simulink library "Source_Lib"  (R2021a)
settings: Solver=VariableStepAuto  StartTime=0.0  StopTime=10.0  RelTol=1e-3
undefined symbols (not defined in the file or in its folder): Cmu0, delta0, fb, GOV1_K2, ia0, ib0, ic0, pha0, phb0, phc0, Theta0_deg, Time_Step, V0_pu, Vfu0
libraries: spsBreakerLib x12, spsControlledVoltageSourceLib x6, spsThreePhaseSourceLib x5, Control_Lib x4, spsThreePhaseVIMeasurementLib x3, spsSeriesRLCBranchLib x2, spsDCVoltageSourceLib x2, spsGroundLib x2, spsLoadFlowBusLib x2, spsThreePhaseParallelRLCLoadLib x1, spsThreePhaseTransformerTwoWindingsLib x1, spsPower3phInstantaneousLib x1
(part 2 of 2)

== system Source_Lib/Generic Voltage Source old/Source_For_OP ==
  v_abc_ref : Inport
  Controlled Voltage Source1 : spsControlledVoltageSourceLib/Controlled Voltage Source  Initialize=off  Source_Type=AC  Amplitude=V0*Ub*sqrt(2/3)*sin(Theta0)  Phase=(Theta0*180/pi)  Frequency=fb  Measurements=None
  Controlled Voltage Source2 : spsControlledVoltageSourceLib/Controlled Voltage Source  Initialize=off  Source_Type=AC  Amplitude=V0*Ub*sqrt(2/3)*sin(Theta0-2*pi/3)  Phase=(Theta0*180/pi)-120  Frequency=fb  Measurements=None
  Controlled Voltage Source3 : spsControlledVoltageSourceLib/Controlled Voltage Source  Initialize=off  Source_Type=AC  Amplitude=V0*Ub*sqrt(2/3)*sin(Theta0-4*pi/3)  Phase=(Theta0*180/pi)+120  Frequency=fb  Measurements=None
  Demux : Demux  Outputs=3
  Step : Step  Time=1e-9  SampleTime=0
  Subsystem3 : Subsystem
  Three-Phase Source1 : spsThreePhaseSourceLib/Three-Phase Source  InternalConnection=Yn  VoltagePhases=off  Voltage=V0_pu*Ub  PhaseAngle=Theta0_deg  Voltage_phases=[25e3 25e3 25e3]/sqrt(3)  PhaseAngles_phases=[0 -120 +120]  Frequency=fb  NonIdealSource=off  SpecifyImpedance=off  Resistance=0.8929  Inductance=16.58e-3  ShortCircuitLevel=100e6  BaseVoltage=25e3  XRratio=7  BusType=swing  Pref=10e3  Qref=0  Prefabc=[10e3, 10e3, 10e3]  Qrefabc=[0, 0, 0]  Qmin=-inf  Qmax=inf
  A : PMIOPort  Side=Right
  B : PMIOPort  Port=2  Side=Right
  C : PMIOPort  Port=3  Side=Right
  N : PMIOPort  Port=4  Side=Left
  wires:
  Demux/2 -> Controlled Voltage Source2/1
  v_abc_ref/1 -> Demux/1
  Demux/1 -> Controlled Voltage Source1/1
  Demux/3 -> Controlled Voltage Source3/1
  Step/1 -> Subsystem3/1(switch)
  connections:
  Controlled Voltage Source3/LConn1 -- Three-Phase Source1/LConn1 -- N/RConn1 -- Controlled Voltage Source2/LConn1 -- Controlled Voltage Source1/LConn1
  Subsystem3/RConn1 -- A/RConn1
  Subsystem3/RConn2 -- B/RConn1
  Subsystem3/RConn3 -- C/RConn1
  Controlled Voltage Source1/RConn1 -- Subsystem3/LConn1
  Controlled Voltage Source2/RConn1 -- Subsystem3/LConn2
  Controlled Voltage Source3/RConn1 -- Subsystem3/LConn3
  Three-Phase Source1/RConn1 -- Subsystem3/LConn4
  Three-Phase Source1/RConn2 -- Subsystem3/LConn5
  Three-Phase Source1/RConn3 -- Subsystem3/LConn6

== system Source_Lib/Synchronous Machine with control and transformer/EX ==
  OP_Vfu : Inport
  Vtdq : Inport  Port=2
  Vref : Inport  Port=3
  vstab : Inport  Port=4
  Filter : Subsystem  mask{K=1, tau=ST1_taur, init_value=V0}
      mask prompts: K "Gain"; tau "Time Constant"; init_value "Initial Value"
  Gain : Gain  Gain=ST1_Ka
  Gain1 : Gain  Gain=1/ST1_Ka
  Module1 : Subsystem
  Sum : Sum  Inputs=+-+-
  Vfu : Outport
  wires:
  Module1/1(||x||) -> Filter/1(In1)
  Filter/1(Output) -> Sum/2
  Vref/1 -> Sum/3
  OP_Vfu/1 -> Gain1/1
  Sum/1 -> Gain/1
  Gain1/1 -> Sum/1
  Vtdq/1 -> Module1/1(x)
  vstab/1 -> Sum/4
  Gain/1 -> Vfu/1

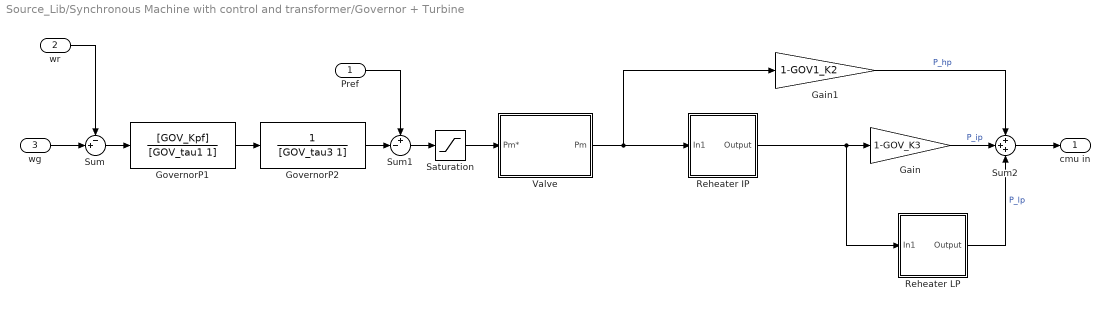
== system Source_Lib/Synchronous Machine with control and transformer/Governor + Turbine ==
  Pref : Inport
  wr : Inport  Port=2
  wg : Inport  Port=3
  Gain : Gain  Gain=1-GOV_K3
  Gain1 : Gain  Gain=1-GOV1_K2
  GovernorP1 : TransferFcn  Numerator=[GOV_Kpf]  Denominator=[GOV_tau1 1]
  GovernorP2 : TransferFcn  Denominator=[GOV_tau3 1]
  Reheater IP : Subsystem  mask{K=GOV_K2, tau=GOV_tau5, init_value=Cmu0*GOV_K2}
      mask prompts: K "Gain"; tau "Time Constant"; init_value "Initial Value"
  Reheater LP : Subsystem  mask{K=GOV_K3, tau=GOV_tau6, init_value=Cmu0*GOV_K2*GOV_K3}
      mask prompts: K "Gain"; tau "Time Constant"; init_value "Initial Value"
  Saturation : Saturate  UpperLimit=1  LowerLimit=0
  Sum : Sum  Inputs=-+|
  Sum1 : Sum  Inputs=+-|
  Sum2 : Sum  Inputs=+++
  Valve : Subsystem  mask{K=1, tau=GOV_tau4, init_value=Cmu0}
      mask prompts: K "Gain"; tau "Time Constant"; init_value "Initial Value"
      mask Display: disp('valve')
  cmu in : Outport
  wires:
  wg/1 -> Sum/2
  GovernorP1/1 -> GovernorP2/1
  GovernorP2/1 -> Sum1/2
  Sum/1 -> GovernorP1/1
  Sum2/1 -> cmu in/1
  Valve/1(Pm) -> Gain1/1, Reheater IP/1(In1)
  Reheater IP/1(Output) -> Gain/1, Reheater LP/1(In1)
  Gain/1 -> Sum2/2  "P_ip"
  Gain1/1 -> Sum2/1  "P_hp"
  Reheater LP/1(Output) -> Sum2/3  "P_lp"
  Sum1/1 -> Saturation/1
  wr/1 -> Sum/1
  Saturation/1 -> Valve/1(Pm*)
  Pref/1 -> Sum1/1

== system Source_Lib/Synchronous Machine with control and transformer/PSS ==
  wr : Inport
  Add1 : Sum  Inputs=-+|
  Constant : Constant
  Gain : Gain  Gain=PSS_K
  P : TransferFcn  Denominator=[PSS_tau6 1]
  Phase compensator 1 : TransferFcn  Numerator=[PSS_tau1 1]  Denominator=[PSS_tau2 1]
  Phase compensator 2 : TransferFcn  Numerator=[PSS_tau3 1]  Denominator=[PSS_tau4 1]
  "Washout\t" : TransferFcn  Numerator=[PSS_tau5 0]  Denominator=[PSS_tau5 1]
  vstab : Outport
  wires:
  "Washout\t"/1 -> Phase compensator 1/1
  Add1/1 -> P/1
  Phase compensator 2/1 -> vstab/1
  Gain/1 -> "Washout\t"/1
  Phase compensator 1/1 -> Phase compensator 2/1
  wr/1 -> Add1/1
  P/1 -> Gain/1
  Constant/1 -> Add1/2

== system Source_Lib/Generic Voltage Source/INERTIAL/CosSin ==
  Theta_rad : Inport
  Mux : Mux  Inputs=2
  Trigonometric Function : Trigonometry
  Trigonometric Function1 : Trigonometry  Operator=cos
  CosSinTheta : Outport  VectorParamsAs1DForOutWhenUnconnected=off
  wires:
  Theta_rad/1 -> Trigonometric Function/1, Trigonometric Function1/1
  Trigonometric Function/1 -> Mux/2
  Mux/1 -> CosSinTheta/1
  Trigonometric Function1/1 -> Mux/1

== system Source_Lib/Generic Voltage Source/INERTIAL/NetworkLeadLagTimeConstants ==
  In1 : Inport
  Constant : Constant  Value=P0
  Integrator3 : Integrator  InitialConditionSource=external  InitialCondition=(P0/Sb)*(1-TN/TD)
  Sum1 : Sum
  Sum2 : Sum  Inputs=+-
  Sum3 : Sum  Inputs=-+
  mp1 : Gain  Gain=TN/TD
  mp2 : Gain  Gain=1-TN/TD
  mp3 : Gain  Gain=1/TD
  Out1 : Outport  VectorParamsAs1DForOutWhenUnconnected=off
  wires:
  Sum1/1 -> Out1/1
  mp1/1 -> Sum3/1, Sum1/1
  mp2/1 -> Sum2/1
  In1/1 -> mp2/1, mp1/1
  mp3/1 -> Integrator3/1
  Sum2/1 -> mp3/1
  Constant/1 -> Sum3/2
  Integrator3/1 -> Sum1/2, Sum2/2
  Sum3/1 -> Integrator3/2

== system Source_Lib/Generic Voltage Source/INFINITE/CosSin ==
  Theta_rad : Inport
  Mux : Mux  Inputs=2
  Trigonometric Function : Trigonometry
  Trigonometric Function1 : Trigonometry  Operator=cos
  CosSinTheta : Outport  VectorParamsAs1DForOutWhenUnconnected=off
  wires:
  Theta_rad/1 -> Trigonometric Function/1, Trigonometric Function1/1
  Trigonometric Function/1 -> Mux/2
  Mux/1 -> CosSinTheta/1
  Trigonometric Function1/1 -> Mux/1

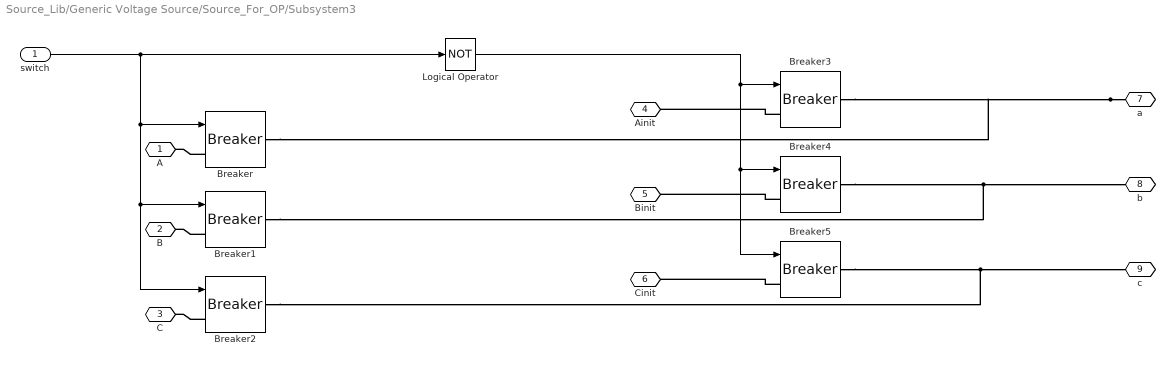
== system Source_Lib/Generic Voltage Source/Source_For_OP/Subsystem3 ==
  switch : Inport
  Breaker : spsBreakerLib/Breaker  InitialState=0  SwitchingTimes="[1/60  5/60]"  External=on  BreakerResistance=0.001  SnubberResistance=1e6  SnubberCapacitance=inf  Measurements=None  MoreParameters=on  NoBreakLoop=off
      settings: SourceProductBaseCode=PS
  Breaker1 : spsBreakerLib/Breaker  InitialState=0  SwitchingTimes="[1/60  5/60]"  External=on  BreakerResistance=0.001  SnubberResistance=1e6  SnubberCapacitance=inf  Measurements=None  MoreParameters=on  NoBreakLoop=off
      settings: SourceProductBaseCode=PS
  Breaker2 : spsBreakerLib/Breaker  InitialState=0  SwitchingTimes="[1/60  5/60]"  External=on  BreakerResistance=0.001  SnubberResistance=1e6  SnubberCapacitance=inf  Measurements=None  MoreParameters=on  NoBreakLoop=off
      settings: SourceProductBaseCode=PS
  Breaker3 : spsBreakerLib/Breaker  InitialState=1  SwitchingTimes="[1/60  5/60]"  External=on  BreakerResistance=0.001  SnubberResistance=1e6  SnubberCapacitance=inf  Measurements=None  MoreParameters=on  NoBreakLoop=off
      settings: SourceProductBaseCode=PS
  Breaker4 : spsBreakerLib/Breaker  InitialState=1  SwitchingTimes="[1/60  5/60]"  External=on  BreakerResistance=0.001  SnubberResistance=1e6  SnubberCapacitance=inf  Measurements=None  MoreParameters=on  NoBreakLoop=off
      settings: SourceProductBaseCode=PS
  Breaker5 : spsBreakerLib/Breaker  InitialState=1  SwitchingTimes="[1/60  5/60]"  External=on  BreakerResistance=0.001  SnubberResistance=1e6  SnubberCapacitance=inf  Measurements=None  MoreParameters=on  NoBreakLoop=off
      settings: SourceProductBaseCode=PS
  Logical Operator : Logic  Operator=NOT  AllPortsSameDT=off  OutDataTypeStr=boolean
  A : PMIOPort  Side=Left
  B : PMIOPort  Port=2  Side=Left
  C : PMIOPort  Port=3  Side=Left
  Ainit : PMIOPort  Port=4  Side=Left
  Binit : PMIOPort  Port=5  Side=Left
  Cinit : PMIOPort  Port=6  Side=Left
  a : PMIOPort  Port=7  Side=Right
  b : PMIOPort  Port=8  Side=Right
  c : PMIOPort  Port=9  Side=Right
  wires:
  Logical Operator/1 -> Breaker3/1, Breaker4/1, Breaker5/1
  switch/1 -> Logical Operator/1, Breaker/1, Breaker1/1, Breaker2/1
  connections:
  Breaker4/RConn1 -- Breaker1/RConn1 -- b/RConn1
  a/RConn1 -- Breaker3/RConn1 -- Breaker/RConn1
  Breaker1/LConn1 -- B/RConn1
  Breaker3/LConn1 -- Ainit/RConn1
  Breaker2/LConn1 -- C/RConn1
  Breaker4/LConn1 -- Binit/RConn1
  Breaker2/RConn1 -- Breaker5/RConn1 -- c/RConn1
  Breaker5/LConn1 -- Cinit/RConn1
  Breaker/LConn1 -- A/RConn1

== system Source_Lib/Generic Voltage Source old/InertialDqVoltageSource/NetworkLeadLagTimeConstants ==
  In1 : Inport
  Integrator3 : Integrator  InitialCondition=(P0/Sb)*(1-TN/TD)
  Sum1 : Sum
  Sum2 : Sum  Inputs=+-
  mp1 : Gain  Gain=TN/TD
  mp2 : Gain  Gain=1-TN/TD
  mp3 : Gain  Gain=1/TD
  Out1 : Outport  VectorParamsAs1DForOutWhenUnconnected=off
  wires:
  Sum1/1 -> Out1/1
  mp1/1 -> Sum1/1
  mp2/1 -> Sum2/1
  In1/1 -> mp2/1, mp1/1
  Integrator3/1 -> Sum2/2, Sum1/2
  mp3/1 -> Integrator3/1
  Sum2/1 -> mp3/1

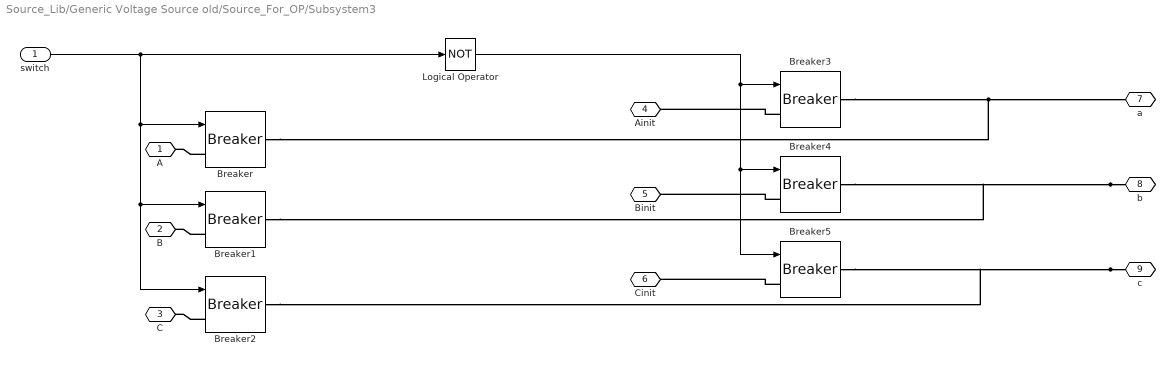
== system Source_Lib/Generic Voltage Source old/Source_For_OP/Subsystem3 ==
  switch : Inport
  Breaker : spsBreakerLib/Breaker  InitialState=0  SwitchingTimes="[1/60  5/60]"  External=on  BreakerResistance=0.001  SnubberResistance=1e6  SnubberCapacitance=inf  Measurements=None  MoreParameters=on  NoBreakLoop=off
      settings: SourceProductBaseCode=PS
  Breaker1 : spsBreakerLib/Breaker  InitialState=0  SwitchingTimes="[1/60  5/60]"  External=on  BreakerResistance=0.001  SnubberResistance=1e6  SnubberCapacitance=inf  Measurements=None  MoreParameters=on  NoBreakLoop=off
      settings: SourceProductBaseCode=PS
  Breaker2 : spsBreakerLib/Breaker  InitialState=0  SwitchingTimes="[1/60  5/60]"  External=on  BreakerResistance=0.001  SnubberResistance=1e6  SnubberCapacitance=inf  Measurements=None  MoreParameters=on  NoBreakLoop=off
      settings: SourceProductBaseCode=PS
  Breaker3 : spsBreakerLib/Breaker  InitialState=1  SwitchingTimes="[1/60  5/60]"  External=on  BreakerResistance=0.001  SnubberResistance=1e6  SnubberCapacitance=inf  Measurements=None  MoreParameters=on  NoBreakLoop=off
      settings: SourceProductBaseCode=PS
  Breaker4 : spsBreakerLib/Breaker  InitialState=1  SwitchingTimes="[1/60  5/60]"  External=on  BreakerResistance=0.001  SnubberResistance=1e6  SnubberCapacitance=inf  Measurements=None  MoreParameters=on  NoBreakLoop=off
      settings: SourceProductBaseCode=PS
  Breaker5 : spsBreakerLib/Breaker  InitialState=1  SwitchingTimes="[1/60  5/60]"  External=on  BreakerResistance=0.001  SnubberResistance=1e6  SnubberCapacitance=inf  Measurements=None  MoreParameters=on  NoBreakLoop=off
      settings: SourceProductBaseCode=PS
  Logical Operator : Logic  Operator=NOT  AllPortsSameDT=off  OutDataTypeStr=boolean
  A : PMIOPort  Side=Left
  B : PMIOPort  Port=2  Side=Left
  C : PMIOPort  Port=3  Side=Left
  Ainit : PMIOPort  Port=4  Side=Left
  Binit : PMIOPort  Port=5  Side=Left
  Cinit : PMIOPort  Port=6  Side=Left
  a : PMIOPort  Port=7  Side=Right
  b : PMIOPort  Port=8  Side=Right
  c : PMIOPort  Port=9  Side=Right
  wires:
  switch/1 -> Breaker2/1, Breaker1/1, Breaker/1, Logical Operator/1
  Logical Operator/1 -> Breaker5/1, Breaker4/1, Breaker3/1
  connections:
  Breaker/LConn1 -- A/RConn1
  Breaker5/LConn1 -- Cinit/RConn1
  c/RConn1 -- Breaker5/RConn1 -- Breaker2/RConn1
  Breaker4/LConn1 -- Binit/RConn1
  Breaker2/LConn1 -- C/RConn1
  Breaker3/LConn1 -- Ainit/RConn1
  Breaker1/LConn1 -- B/RConn1
  Breaker/RConn1 -- Breaker3/RConn1 -- a/RConn1
  b/RConn1 -- Breaker1/RConn1 -- Breaker4/RConn1

== system Source_Lib/Synchronous Machine with control and transformer/EX/Filter ==
  In1 : Inport
  Gain : Gain  Gain=K
  Gain3 : Gain  Gain=1/tau
  Integrator : Integrator  InitialCondition=init_value/K
  Sum3 : Sum  Inputs=|+-
  Output : Outport
  wires:
  In1/1 -> Sum3/1
  Sum3/1 -> Gain3/1
  Integrator/1 -> Sum3/2, Gain/1
  Gain/1 -> Output/1
  Gain3/1 -> Integrator/1

== system Source_Lib/Synchronous Machine with control and transformer/EX/Module1 ==
  x : Inport
  Add1 : Sum
  Demux : Demux  Outputs=2
  Math Function : Math  Operator=square  SaturateOnIntegerOverflow=on
  Math Function1 : Math  Operator=square  SaturateOnIntegerOverflow=on
  Sqrt : Sqrt  SaturateOnIntegerOverflow=on
  ||x|| : Outport
  wires:
  Demux/2 -> Math Function1/1
  Sqrt/1 -> ||x||/1
  x/1 -> Demux/1
  Math Function1/1 -> Add1/2
  Math Function/1 -> Add1/1
  Add1/1 -> Sqrt/1
  Demux/1 -> Math Function/1

== system Source_Lib/Synchronous Machine with control and transformer/Governor + Turbine/Reheater IP ==
  In1 : Inport
  Constant : Constant  Value=init_value/K
  Gain : Gain  Gain=K
  Gain3 : Gain  Gain=1/tau
  Integrator : Integrator  InitialConditionSource=external
  Sum3 : Sum  Inputs=|+-
  Output : Outport
  wires:
  Constant/1 -> Integrator/2
  In1/1 -> Sum3/1
  Sum3/1 -> Gain3/1
  Integrator/1 -> Sum3/2, Gain/1
  Gain/1 -> Output/1
  Gain3/1 -> Integrator/1

== system Source_Lib/Synchronous Machine with control and transformer/Governor + Turbine/Reheater LP ==
  In1 : Inport
  Constant : Constant  Value=init_value/K
  Gain : Gain  Gain=K
  Gain3 : Gain  Gain=1/tau
  Integrator : Integrator  InitialConditionSource=external
  Sum3 : Sum  Inputs=|+-
  Output : Outport
  wires:
  Constant/1 -> Integrator/2
  Gain3/1 -> Integrator/1
  Gain/1 -> Output/1
  Integrator/1 -> Sum3/2, Gain/1
  Sum3/1 -> Gain3/1
  In1/1 -> Sum3/1

== system Source_Lib/Synchronous Machine with control and transformer/Governor + Turbine/Valve ==
  Pm* : Inport
  Constant : Constant  Value=init_value/K
  Gain : Gain  Gain=K
  Gain3 : Gain  Gain=1/tau
  Integrator : Integrator  InitialConditionSource=external
  Sum3 : Sum  Inputs=|+-
  Pm : Outport
  wires:
  Constant/1 -> Integrator/2
  Gain3/1 -> Integrator/1
  Gain/1 -> Pm/1
  Integrator/1 -> Sum3/2, Gain/1
  Sum3/1 -> Gain3/1
  Pm*/1 -> Sum3/1
